simulink model "systems"  (R2019b)
settings: Solver=VariableStepAuto  StartTime=0.0  StopTime=354  RelTol=1e-3
settings Model: Creator=Amir Edge  LastModifiedBy=Amir Edge

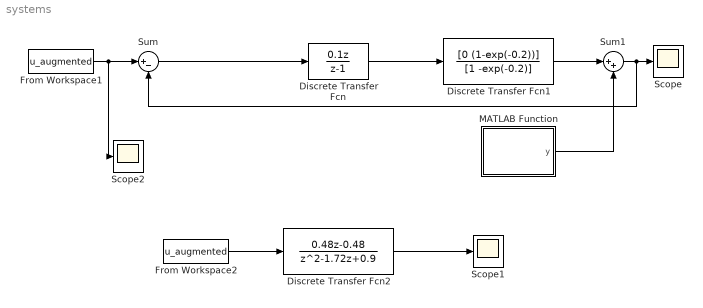
== system systems ==
  Discrete Transfer Fcn : DiscreteTransferFcn  Numerator=[0.1 0]  Denominator=[1 -1]
  Discrete Transfer Fcn1 : DiscreteTransferFcn  Numerator=[0 (1-exp(-0.2))]  Denominator=[1 -exp(-0.2)]
  Discrete Transfer Fcn2 : DiscreteTransferFcn  Numerator=[0.48 -0.48]  Denominator=[1 -1.72 0.9]
  From Workspace1 : FromWorkspace  VariableName=u_augmented  SampleTime=1
  From Workspace2 : FromWorkspace  VariableName=u_augmented  SampleTime=1
  MATLAB Function : MATLAB Function  TreatAsAtomicUnit=on
  Scope : Scope
  Scope1 : Scope
  Scope2 : Scope
  Sum : Sum  Inputs=|+-
  Sum1 : Sum  Inputs=|++
  wires:
  Discrete Transfer Fcn/1 -> Discrete Transfer Fcn1/1
  Sum/1 -> Discrete Transfer Fcn/1
  Discrete Transfer Fcn1/1 -> Sum1/1
  From Workspace1/1 -> Scope2/1, Sum/1
  From Workspace2/1 -> Discrete Transfer Fcn2/1
  Discrete Transfer Fcn2/1 -> Scope1/1
  MATLAB Function/1(y) -> Sum1/2
  Sum1/1 -> Sum/2, Scope/1

== matlab function systems/MATLAB Function ==
  data: y output
function y = fcn()
sigma = 0.01;
mu = 0;
y = normrnd(mu, sigma);
